simulink model "direct_moter_input"  (R2023b)
settings: Solver=FixedStepAuto  StartTime=0.0  StopTime=inf  RelTol=1e-3  EnableMultiTasking=on
undefined symbols (not defined in the file): AUX, dev, pwm_output1
libraries: px4lib x1, px4Sensorslib x1
settings Model: ExtModeTrigDuration=10  Creator=yamak  LastModifiedBy=yamak
settings SolverCC: PositivePriorityOrder=on
settings OptimizationCC: EnhancedBackFolding=on  PassReuseOutputArgsAs=Individual arguments  ZeroExternalMemoryAtStartup=off  ZeroInternalMemoryAtStartup=off  MaxStackSize=64  OptimizeBlockOrder=speed  DifferentSizesBufferReuse=on  OptimizationCustomize=off  EfficientTunableParamExpr=on
settings DebuggingCC: ParameterTunabilityLossMsg=error
settings HardwareCC: ProdBitPerPointer=32  ProdBitPerSizeT=32  ProdBitPerPtrDiffT=32  ProdLargestAtomicInteger=Long  ProdLargestAtomicFloat=Double  ProdWordSize=32  ProdLongLongMode=on  ProdHWDeviceType=ARM Compatible->ARM Cortex
settings SFSimCC: MATLABDynamicMemAlloc=off  SimTargetLang=C++
settings RTWCC: Description=Embedded Coder  SystemTargetFile=ert.tlc  HardwareBoard=PX4 Pixhawk 4  TLCOptions="-aInlineSetEventsForThisBaseRateFcn=TLC_FALSE -aSuppressMultiTaskScheduler=TLC_FALSE  -aRateBasedStepFcn=0"  TemplateMakefile=ert_default_tmf  Toolchain=GNU Tools for PX4 Autopilots  TargetLang=C++
settings CodeAppCC: ForceParamTrailComments=on  IgnoreCustomStorageClasses=off  OperatorAnnotations=on  SimulinkDataObjDesc=on  SFDataObjDesc=on  InsertBlockDesc=on
settings ERTTargetCC: ExtModeTransport=3  ExtModeStaticAlloc=on  ExtModeStaticAllocSize=1024  ExtModeMexFile=ext_xcp  ExtModeIntrfLevel=Level2 - Open

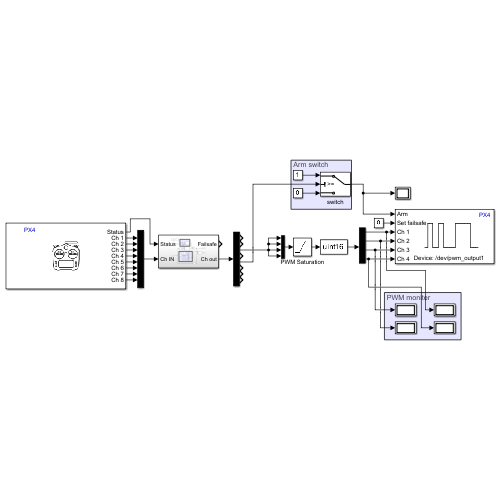
[thumbnail: Simulink's stored preview of the top-level diagram]
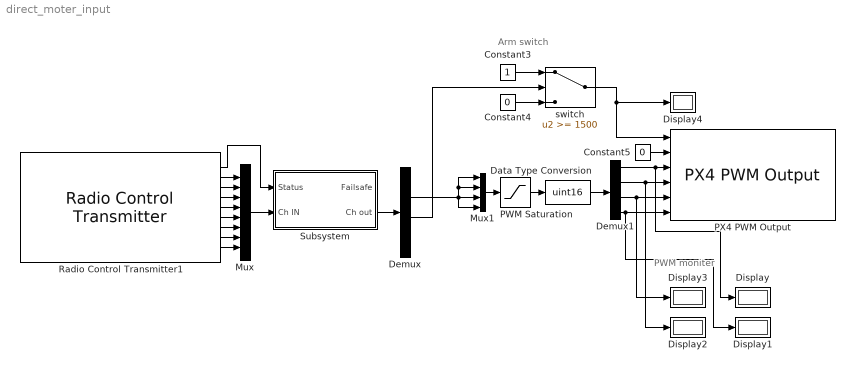
== system direct_moter_input ==
  note: PWM moniter
  note: Arm switch
  Constant3 : Constant  OutDataTypeStr=boolean
  Constant4 : Constant  Value=0  OutDataTypeStr=boolean
  Constant5 : Constant  Value=0  OutDataTypeStr=boolean
  Data Type Conversion : DataTypeConversion  OutDataTypeStr=uint16  SaturateOnIntegerOverflow=off  RndMeth=Floor
  Demux : Demux  Outputs=8
  Demux1 : Demux
  Display{,1..4} (5 alike) : Display
  Mux : Mux  Inputs=8
  Mux1 : Mux
  PWM Saturation : Saturate  UpperLimit=2000  LowerLimit=1000
  PX4 PWM Output : px4lib/PX4 PWM Output  pwmDevice=AUX (/dev/pwm_output1)  pwmChannel1_=on  pwmChannel2_=on  pwmChannel3_=on  pwmChannel4_=on  pwmChannel5_=off  pwmChannel6_=off  pwmChannel7_=off  pwmChannel8_=off  forceTerminateFailsafe=off  outputErrorStatus=off
  Radio Control Transmitter1 : px4Sensorslib/Radio Control Transmitter  channel1=on  channel2=on  channel3=on  channel4=on  channel5=on  channel6=on  channel7=on  channel8=on  channel_count=off  rssi=off  rc_input_source=off  timestamp_last_signal=off  time_stamp=off  sampleTime=1/250  BlockingMode=off  BlockTimeout=5
  Subsystem : Subsystem
  switch : Switch  Threshold=1500  OutDataTypeStr=boolean  SaturateOnIntegerOverflow=off  InputSameDT=off
  wires:
  Radio Control Transmitter1/5 -> Mux/4
  Radio Control Transmitter1/1 -> Subsystem/1(Status)
  Radio Control Transmitter1/8 -> Mux/7
  Mux/1 -> Subsystem/2(Ch IN)
  Radio Control Transmitter1/7 -> Mux/6
  Radio Control Transmitter1/6 -> Mux/5
  Radio Control Transmitter1/2 -> Mux/1
  Radio Control Transmitter1/4 -> Mux/3
  Radio Control Transmitter1/3 -> Mux/2
  Subsystem/2(Ch out) -> Demux/1
  Constant5/1 -> PX4 PWM Output/2
  switch/1 -> Display4/1, PX4 PWM Output/1
  Demux1/1 -> Display/1, PX4 PWM Output/3
  Demux1/3 -> PX4 PWM Output/5, Display3/1
  Demux1/2 -> PX4 PWM Output/4, Display2/1
  Demux1/4 -> Display1/1, PX4 PWM Output/6
  PWM Saturation/1 -> Data Type Conversion/1
  Data Type Conversion/1 -> Demux1/1
  Constant4/1 -> switch/3
  Constant3/1 -> switch/1
  Demux/5 -> switch/2
  Demux/3 -> Mux1/4, Mux1/1, Mux1/2, Mux1/3
  Mux1/1 -> PWM Saturation/1
  Radio Control Transmitter1/9 -> Mux/8

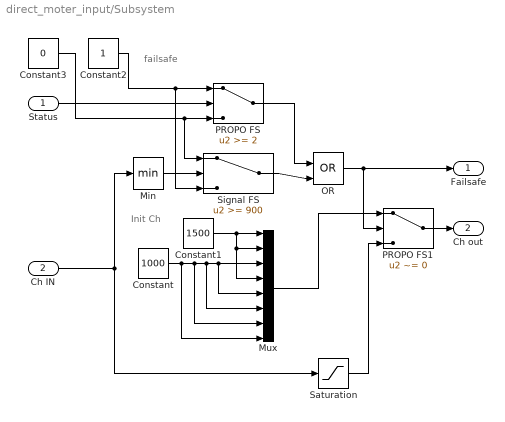
== system direct_moter_input/Subsystem ==
  note: Init Ch
  note: failsafe
  Status : Inport
  Ch IN : Inport  Port=2
  Constant : Constant  Value=1000
  Constant1 : Constant  Value=1500
  Constant2 : Constant  OutDataTypeStr=boolean
  Constant3 : Constant  Value=0  OutDataTypeStr=boolean
  Min : MinMax
  Mux : Mux  Inputs=8
  OR : Logic  Operator=OR  IconShape=distinctive  AllPortsSameDT=off  OutDataTypeStr=boolean
  PROPO FS : Switch  Threshold=2  OutDataTypeStr=boolean  SaturateOnIntegerOverflow=off  InputSameDT=off
  PROPO FS1 : Switch  Criteria=u2 ~= 0  Threshold=2  SaturateOnIntegerOverflow=off  InputSameDT=off
  Saturation : Saturate  UpperLimit=2000  LowerLimit=1000
  Signal FS : Switch  Threshold=900  OutDataTypeStr=boolean  SaturateOnIntegerOverflow=off  InputSameDT=off
  Failsafe : Outport
  Ch out : Outport  Port=2
  wires:
  Constant1/1 -> Mux/1, Mux/4, Mux/2
  Constant/1 -> Mux/8, Mux/7, Mux/6, Mux/5, Mux/3
  Constant3/1 -> Signal FS/1, PROPO FS/3
  PROPO FS/1 -> OR/1
  Ch IN/1 -> Min/1, Saturation/1
  Mux/1 -> PROPO FS1/1
  PROPO FS1/1 -> Ch out/1
  OR/1 -> Failsafe/1, PROPO FS1/2
  Status/1 -> PROPO FS/2
  Min/1 -> Signal FS/2
  Constant2/1 -> PROPO FS/1, Signal FS/3
  Signal FS/1 -> OR/2
  Saturation/1 -> PROPO FS1/3
